simulink model "Monotonic_test"  (Simulink 7.3)
settings: Solver=ode45  StartTime=0.0  StopTime=10.0  RelTol=1e-3
settings Model: Creator=MD710  LastModifiedBy=MD710
settings DebuggingCC: SaveWithParameterizedLinksMsg=none  SolverPrmCheckMsg=none  MultiTaskDSMMsg=warning  MultiTaskCondExecSysMsg=none  FcnCallInpInsideContextMsg=Enable All  StrictBusMsg=None
settings HardwareCC: TargetHWDeviceType=32-bit Generic
settings RTWCC: IncludeERTFirstTime=on
settings GRTTargetCC: TargetFcnLib=ansi_tfl_tmw.mat

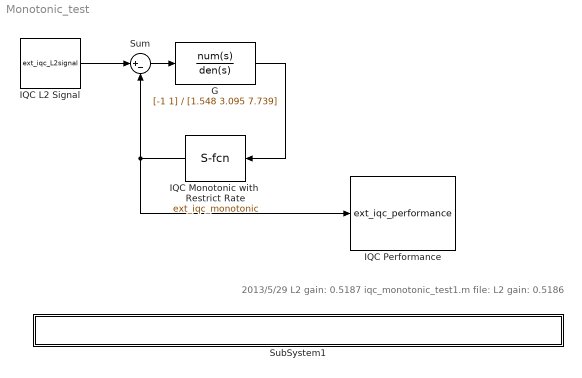
== system Monotonic_test ==
  note: 2013/5/29 L2 gain: 0.5187
      | iqc_monotonic_test1.m file: L2 gain: 0.5186
  G : TransferFcn  Numerator=[-1 1]  Denominator=[1.548 3.095 7.739]
  IQC L2 Signal : M-S-Function  FunctionName=ext_iqc_L2signal  Parameters=sig_size,sam_time,sig_type,tru_time,sig_amp,sig_fre,user_cus  mask(IQC L2 signal(ver:0.1)){sig_size=1, sam_time=0, sig_type=Step, tru_time=10, sig_amp=1, sig_fre=1, user_cus='2*exp(3*t)'}
      mask prompts: sig_size "Signal Dimension:(Default: 1)"; sam_time "Sample Time:(Default: 0)"; sig_type "Signal Type:"; tru_time "Truncation Time:"; sig_amp "Maximum Amplitude:"; sig_fre "Frequency:"; user_cus "Custom:"
      mask help:
      | Important:
      | In IQC procedure step (as commond iqc_gain_tbx, the task is get
      | L2 gain value), regardless of the user to choose which option (ex sine...),
      | here regarded as generalized L2 signal.
      mask StyleString: edit,edit,popup(Step|Square wave|Sine wave|Custom|Random|External),edit,edit,edit,edit
      mask CallbackString: ||iqc_block_cho(gcb,'L2signal_type')||||
      mask TabNameString: Generalized Parameters,Generalized Parameters,Simulink Parameters,Simulink Parameters,Simulink Parameters,Simulink Parameters,Simulink Parameters
      mask Display: plot(0:0.1:10,[sin(0:0.1:6.2) zeros(1,38)])
  IQC Monotonic with  Restrict Rate : M-S-Function  FunctionName=ext_iqc_monotonic  Parameters=pole,int_dd,ope,out_var  mask(IQC Monotonic with Restrict Rate(ver:0.1)){pole=[1], ope=0 (shut off the Popov's IQC), int_dd=1, out_var=''}
      mask prompts: pole "Pole:(Default: [1])"; ope "Operator:(Default: 0)"; int_dd "Interval of d(delta)/dt:(Default: 1)"; out_var "Output Variable:(Default: empty)"
      mask help:
      | Example: [w,xa,xb,xc,xd,xpop]=iqc_monotonic(v,a,op,k)
      | Pole:
      |          [a]
      | Operator:
      |          [op]
      | Interval of d(delta)/dt:
      |          [k]
      | Output Variable:
      |          {'xa','xb','xc','xd','xpop'}
      mask Help: eval('doc iqc_monotonic')
      mask StyleString: edit,popup(0 (shut off the Popov's IQC)|1 (turn on the Popov's IQC)),edit,edit
      mask Display: plot(0,0,100,100,[99,-0],[50,50],[50,50],[-0,100],[10,90],[0,100],[99,95,88,82,75,70,67,60,55,50],[76,76,75,74,72,70,68,62,56,50],[1,5,9,16,22,29,34,40,45,50],[20,21,22,24,26,29,32,38,44,50]);
  IQC Performance : M-S-Function  FunctionName=ext_iqc_performance  Parameters=imp_met,save_lin_com,isiqcbode,fre_ran,uselmitool,lmi_par  mask(IQC Performance(ver:0.1)){imp_met=Only Calculation, save_lin_com=off, isiqcbode=off, fre_ran='', uselmitool=lmilab, lmi_par=''}
      mask prompts: imp_met "Implementation Methods"; save_lin_com "Save the Linear File and Command File"; isiqcbode "Display IQC Bode Figure"; fre_ran "Frequency Range:(Default: empty)"; uselmitool "LMI Tool:"; lmi_par "Parameter:(if empty use define)"
      mask help:
      | Important:
      | In IQC toolbox calculate step (as commond iqc_gain_tbx, the task is get
      | L2 gain value), regardless of the user to connect any signal input(Even if
      | not a signal), here regarded as generalized L2 signal.
      |
      | Example 1: setlmioptions('',[0 200 0 0 777])
      | the block parameter is
      | LMI Tool: lmilab
      | Parameter:
      |        [0 200 0 0 777]
      |
      | Example 2: setlmioptions('yalmip','solver','sdpt3','verbose',1)
      | the block parameter is
      | LMI Tool: yalmip
      | Parameter:
      |        {'solver',sdpt3','verbose',1}
      mask Help:
      | <a href="matlab:doc abst_init_iqc;">abst_init_iqc</a>
      | <a href="matlab:doc setlmioptions;">setlmioptions</a>
      | <a href="matlab:doc iqc_gain_tbx;">iqc_gain_tbx</a>
      mask StyleString: popup(Calculation and Simulation|Only Calculation|Only Simulation),checkbox,checkbox,edit,popup(lmilab|yalmip),edit
      mask CallbackString: iqc_block_cho(gcb,'performance_imp')||iqc_block_cho(gcb,'performance_bodefre')|||
      mask TabNameString: Parameter,Parameter,Parameter,Parameter,LMI Parameter,LMI Parameter
      mask Display: fprintf('In -> Out \n performance \n L2 gain:\n%4.4f',0.51869);
  SubSystem1 : Subsystem  mask{filename=iqc_monotonic_test1.m}
      mask init:
      | x_dir=which(filename);
      | x=x_dir;
      settings: OpenFcn=|
      | x_dir=which('iqc_monotonic_test1.m');
      | x=x_dir;
      | edit(x);
      mask Display: disp(['MATLAB file: ' x]);
  Sum : Sum  Inputs=|+-
  wires:
  Sum/1 -> G/1
  IQC L2 Signal/1 -> Sum/1
  G/1 -> IQC Monotonic with  Restrict Rate/1
  IQC Monotonic with  Restrict Rate/1 -> IQC Performance/1, Sum/2

== system Monotonic_test/SubSystem1 ==
